simulink model "fas3dboc_2dexp_2019a"  (R2019a)
settings: Solver=ode4  StartTime=0.0  StopTime=20  FixedStep=0.1  RelTol=1e-3
libraries: sldrtlib x1
settings Model: Creator=star-laptop  LastModifiedBy=nochinese
settings DebuggingCC: UnconnectedInputMsg=none  UnconnectedOutputMsg=none  UnconnectedLineMsg=none

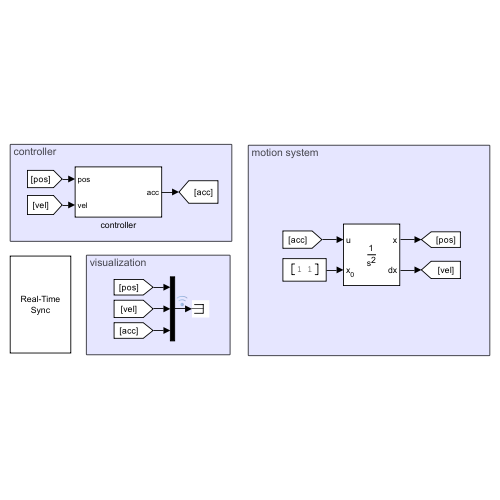
[thumbnail: Simulink's stored preview of the top-level diagram]
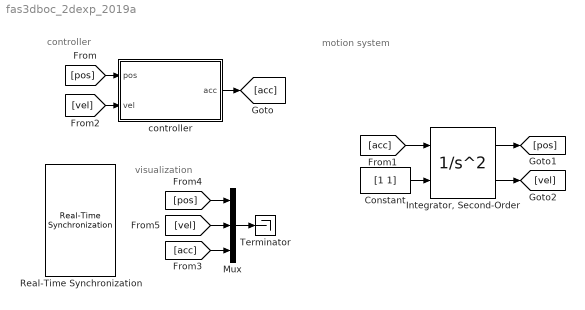
== system fas3dboc_2dexp_2019a ==
  note: motion system
  note: controller
  note: visualization
  Constant : Constant  Value=[1 1]
  "Integrator, Second-Order" : SecondOrderIntegrator  ICSourceX=external
  Mux : Mux  Inputs=3
  Real-Time Synchronization : sldrtlib/Real-Time Synchronization  SampleTime=0.1  MaxMissedTicks=10  ShowMissedTicks=off  YieldWhenWaiting=off
  Terminator : Terminator
  controller : Subsystem
  wires:
  controller/1(acc) -> [acc]
  [pos] -> controller/1(pos)
  "Integrator, Second-Order"/1 -> [pos]
  [acc] -> "Integrator, Second-Order"/1
  Constant/1 -> "Integrator, Second-Order"/2
  "Integrator, Second-Order"/2 -> [vel]
  [vel] -> controller/2(vel)
  Mux/1 -> Terminator/1
  [acc] -> Mux/3
  [pos] -> Mux/1
  [vel] -> Mux/2

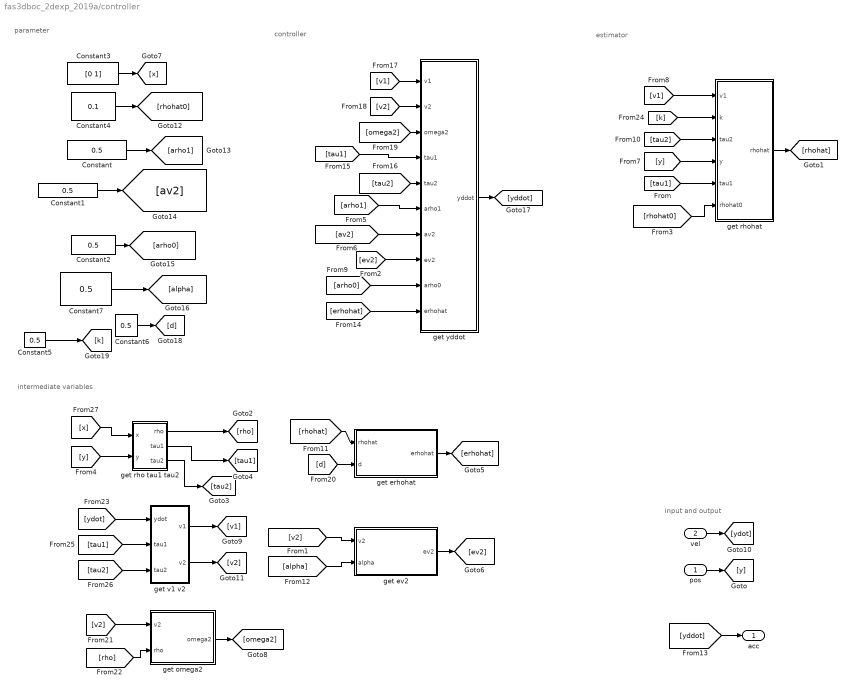
== system fas3dboc_2dexp_2019a/controller ==
  note: intermediate variables
  note: estimator
  note: controller
  note: parameter
  note: input and output
  pos : Inport
  vel : Inport  Port=2
  Constant{,1..2,5..7} (6 alike) : Constant  Value=0.5
  Constant3 : Constant  Value=[0 1]
  Constant4 : Constant  Value=0.1
  get erhohat : Subsystem
  get ev2 : Subsystem
  get omega2 : Subsystem
  get rho tau1 tau2 : Subsystem
  get rhohat : Subsystem
  get v1 v2 : Subsystem
  get yddot : Subsystem
  acc : Outport
  wires:
  pos/1 -> [y]
  [v1] -> get rhohat/1(v1)
  [tau2] -> get rhohat/3(tau2)
  [y] -> get rhohat/4(y)
  [tau1] -> get rhohat/5(tau1)
  get rhohat/1(rhohat) -> [rhohat]
  [rhohat] -> get erhohat/1(rhohat)
  get erhohat/1(erhohat) -> [erhohat]
  [v1] -> get yddot/1(v1)
  [v2] -> get yddot/2(v2)
  [omega2] -> get yddot/3(omega2)
  [tau1] -> get yddot/4(tau1)
  [tau2] -> get yddot/5(tau2)
  [ev2] -> get yddot/8(ev2)
  [erhohat] -> get yddot/10(erhohat)
  [v2] -> get ev2/1(v2)
  get ev2/1(ev2) -> [ev2]
  Constant3/1 -> [x]
  [v2] -> get omega2/1(v2)
  [rho] -> get omega2/2(rho)
  get omega2/1(omega2) -> [omega2]
  [ydot] -> get v1 v2/1(ydot)
  [tau1] -> get v1 v2/2(tau1)
  [tau2] -> get v1 v2/3(tau2)
  get v1 v2/1(v1) -> [v1]
  get v1 v2/2(v2) -> [v2]
  vel/1 -> [ydot]
  [x] -> get rho tau1 tau2/1(x)
  [y] -> get rho tau1 tau2/2(y)
  get rho tau1 tau2/1(rho) -> [rho]
  get rho tau1 tau2/2(tau1) -> [tau1]
  get rho tau1 tau2/3(tau2) -> [tau2]
  Constant4/1 -> [rhohat0]
  [rhohat0] -> get rhohat/6(rhohat0)
  Constant/1 -> [arho1]
  [arho1] -> get yddot/6(arho1)
  Constant1/1 -> [av2]
  [arho0] -> get yddot/9(arho0)
  Constant2/1 -> [arho0]
  [av2] -> get yddot/7(av2)
  [d] -> get erhohat/2(d)
  Constant6/1 -> [d]
  Constant7/1 -> [alpha]
  [alpha] -> get ev2/2(alpha)
  [yddot] -> acc/1
  get yddot/1(yddot) -> [yddot]
  Constant5/1 -> [k]
  [k] -> get rhohat/2(k)

== system fas3dboc_2dexp_2019a/controller/get erhohat ==
  rhohat : Inport
  d : Inport  Port=2
  Subtract : Sum  Inputs=+-
  erhohat : Outport
  wires:
  rhohat/1 -> Subtract/1
  d/1 -> Subtract/2
  Subtract/1 -> erhohat/1

== system fas3dboc_2dexp_2019a/controller/get ev2 ==
  v2 : Inport
  alpha : Inport  Port=2
  Subtract : Sum  Inputs=+-
  ev2 : Outport
  wires:
  v2/1 -> Subtract/1
  alpha/1 -> Subtract/2
  Subtract/1 -> ev2/1

== system fas3dboc_2dexp_2019a/controller/get omega2 ==
  v2 : Inport
  rho : Inport  Port=2
  Divide : Product  Inputs=*/
  omega2 : Outport
  wires:
  v2/1 -> Divide/1
  rho/1 -> Divide/2
  Divide/1 -> omega2/1

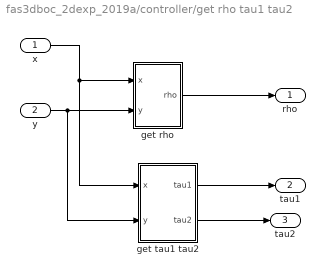
== system fas3dboc_2dexp_2019a/controller/get rho tau1 tau2 ==
  x : Inport
  y : Inport  Port=2
  get rho : Subsystem
  get tau1 tau2 : Subsystem
  rho : Outport
  tau1 : Outport  Port=2
  tau2 : Outport  Port=3
  wires:
  get tau1 tau2/2(tau2) -> tau2/1
  y/1 -> get tau1 tau2/2(y), get rho/2(y)
  get rho/1(rho) -> rho/1
  x/1 -> get tau1 tau2/1(x), get rho/1(x)
  get tau1 tau2/1(tau1) -> tau1/1

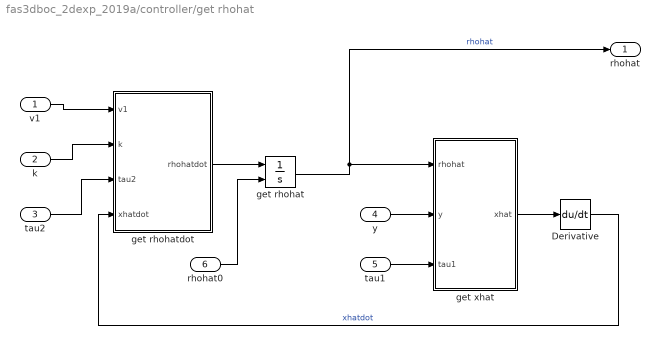
== system fas3dboc_2dexp_2019a/controller/get rhohat ==
  v1 : Inport
  k : Inport  Port=2
  tau2 : Inport  Port=3
  y : Inport  Port=4
  tau1 : Inport  Port=5
  rhohat0 : Inport  Port=6
  Derivative : Derivative
  get rhohat : Integrator  InitialConditionSource=external
  get rhohatdot : Subsystem
  get xhat : Subsystem
  rhohat : Outport
  wires:
  y/1 -> get xhat/2(y)
  get rhohat/1 -> rhohat/1, get xhat/1(rhohat)  "rhohat"
  get xhat/1(xhat) -> Derivative/1
  tau2/1 -> get rhohatdot/3(tau2)
  Derivative/1 -> get rhohatdot/4(xhatdot)  "xhatdot"
  get rhohatdot/1(rhohatdot) -> get rhohat/1
  v1/1 -> get rhohatdot/1(v1)
  tau1/1 -> get xhat/3(tau1)
  k/1 -> get rhohatdot/2(k)
  rhohat0/1 -> get rhohat/2

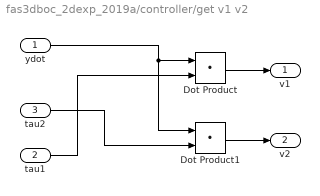
== system fas3dboc_2dexp_2019a/controller/get v1 v2 ==
  ydot : Inport
  tau1 : Inport  Port=2
  tau2 : Inport  Port=3
  Dot Product : DotProduct  InputSameDT=on  OutDataTypeStr=Inherit: Inherit via internal rule
  Dot Product1 : DotProduct  InputSameDT=on  OutDataTypeStr=Inherit: Inherit via internal rule
  v1 : Outport
  v2 : Outport  Port=2
  wires:
  ydot/1 -> Dot Product1/1, Dot Product/1
  Dot Product/1 -> v1/1
  Dot Product1/1 -> v2/1
  tau2/1 -> Dot Product1/2
  tau1/1 -> Dot Product/2

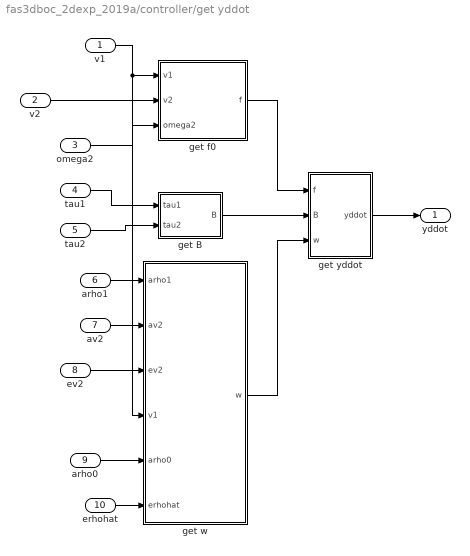
== system fas3dboc_2dexp_2019a/controller/get yddot ==
  v1 : Inport
  v2 : Inport  Port=2
  omega2 : Inport  Port=3
  tau1 : Inport  Port=4
  tau2 : Inport  Port=5
  arho1 : Inport  Port=6
  av2 : Inport  Port=7
  ev2 : Inport  Port=8
  arho0 : Inport  Port=9
  erhohat : Inport  Port=10
  get B : Subsystem
  get f0 : Subsystem
  get w : Subsystem
  get yddot : Subsystem
  yddot : Outport
  wires:
  tau1/1 -> get B/1(tau1)
  get B/1(B) -> get yddot/2(B)
  av2/1 -> get w/2(av2)
  ev2/1 -> get w/3(ev2)
  get yddot/1(yddot) -> yddot/1
  v1/1 -> get w/4(v1), get f0/1(v1)
  get w/1(w) -> get yddot/3(w)
  get f0/1(f) -> get yddot/1(f)
  v2/1 -> get f0/2(v2)
  omega2/1 -> get f0/3(omega2)
  tau2/1 -> get B/2(tau2)
  arho1/1 -> get w/1(arho1)
  erhohat/1 -> get w/6(erhohat)
  arho0/1 -> get w/5(arho0)

== system fas3dboc_2dexp_2019a/controller/get rho tau1 tau2/get rho ==
  note: $\rho=\|{\bf\it x}-{\bf\it y}\|$
  x : Inport
  y : Inport  Port=2
  Add : Sum  Inputs=+-
  Dot Product : DotProduct  InputSameDT=on  OutDataTypeStr=Inherit: Inherit via internal rule
  Sqrt : Sqrt  SaturateOnIntegerOverflow=on
  rho : Outport
  wires:
  Dot Product/1 -> Sqrt/1
  Add/1 -> Dot Product/2, Dot Product/1
  y/1 -> Add/2
  x/1 -> Add/1
  Sqrt/1 -> rho/1

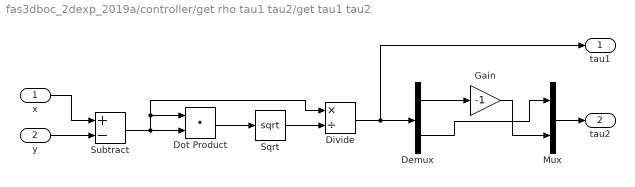
== system fas3dboc_2dexp_2019a/controller/get rho tau1 tau2/get tau1 tau2 ==
  x : Inport
  y : Inport  Port=2
  Demux : Demux  Outputs=2
  Divide : Product  Inputs=*/
  Dot Product : DotProduct  InputSameDT=on  OutDataTypeStr=Inherit: Inherit via internal rule
  Gain : Gain  Gain=-1
  Mux : Mux  Inputs=2
  Sqrt : Sqrt  SaturateOnIntegerOverflow=on
  Subtract : Sum  Inputs=+-
  tau1 : Outport
  tau2 : Outport  Port=2
  wires:
  Divide/1 -> tau1/1, Demux/1
  y/1 -> Subtract/2
  Sqrt/1 -> Divide/2
  Dot Product/1 -> Sqrt/1
  Gain/1 -> Mux/2
  Demux/2 -> Mux/1
  Subtract/1 -> Divide/1, Dot Product/1, Dot Product/2
  Demux/1 -> Gain/1
  Mux/1 -> tau2/1
  x/1 -> Subtract/1

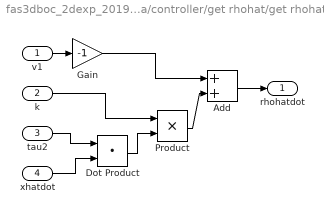
== system fas3dboc_2dexp_2019a/controller/get rhohat/get rhohatdot ==
  v1 : Inport
  k : Inport  Port=2
  tau2 : Inport  Port=3
  xhatdot : Inport  Port=4
  Add : Sum
  Dot Product : DotProduct  InputSameDT=on  OutDataTypeStr=Inherit: Inherit via internal rule
  Gain : Gain  Gain=-1
  Product : Product
  rhohatdot : Outport
  wires:
  tau2/1 -> Dot Product/1
  xhatdot/1 -> Dot Product/2
  Dot Product/1 -> Product/2
  k/1 -> Product/1
  v1/1 -> Gain/1
  Product/1 -> Add/2
  Gain/1 -> Add/1
  Add/1 -> rhohatdot/1

== system fas3dboc_2dexp_2019a/controller/get rhohat/get xhat ==
  rhohat : Inport
  y : Inport  Port=2
  tau1 : Inport  Port=3
  Add : Sum
  Product : Product
  xhat : Outport
  wires:
  rhohat/1 -> Product/1
  tau1/1 -> Product/2
  y/1 -> Add/1
  Product/1 -> Add/2
  Add/1 -> xhat/1

== system fas3dboc_2dexp_2019a/controller/get yddot/get B ==
  tau1 : Inport
  tau2 : Inport  Port=2
  Gain : Gain  Gain=-1
  Matrix Concatenate : Concatenate  Mode=Multidimensional array  ConcatenateDimension=2
  Transpose : Math  Operator=transpose  SaturateOnIntegerOverflow=on
  B : Outport
  wires:
  tau1/1 -> Gain/1
  Gain/1 -> Matrix Concatenate/1
  tau2/1 -> Matrix Concatenate/2
  Matrix Concatenate/1 -> Transpose/1
  Transpose/1 -> B/1

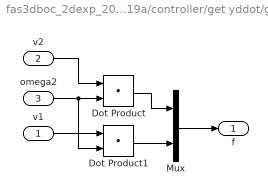
== system fas3dboc_2dexp_2019a/controller/get yddot/get f0 ==
  v1 : Inport
  v2 : Inport  Port=2
  omega2 : Inport  Port=3
  Dot Product : DotProduct  InputSameDT=on  OutDataTypeStr=Inherit: Inherit via internal rule
  Dot Product1 : DotProduct  InputSameDT=on  OutDataTypeStr=Inherit: Inherit via internal rule
  Mux : Mux  Inputs=2
  f : Outport
  wires:
  Dot Product1/1 -> Mux/2
  v2/1 -> Dot Product/1
  Mux/1 -> f/1
  omega2/1 -> Dot Product1/2, Dot Product/2
  v1/1 -> Dot Product1/1
  Dot Product/1 -> Mux/1

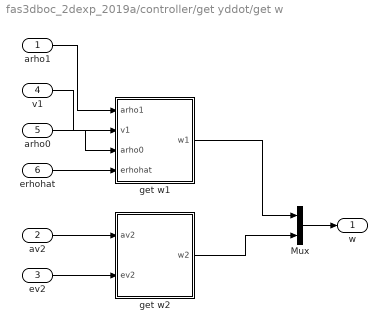
== system fas3dboc_2dexp_2019a/controller/get yddot/get w ==
  arho1 : Inport
  av2 : Inport  Port=2
  ev2 : Inport  Port=3
  v1 : Inport  Port=4
  arho0 : Inport  Port=5
  erhohat : Inport  Port=6
  Mux : Mux  Inputs=2
  get w1 : Subsystem
  get w2 : Subsystem
  w : Outport
  wires:
  get w1/1(w1) -> Mux/1
  Mux/1 -> w/1
  av2/1 -> get w2/1(av2)
  ev2/1 -> get w2/2(ev2)
  erhohat/1 -> get w1/4(erhohat)
  arho0/1 -> get w1/3(arho0)
  v1/1 -> get w1/2(v1)
  arho1/1 -> get w1/1(arho1)
  get w2/1(w2) -> Mux/2

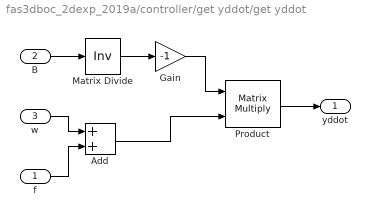
== system fas3dboc_2dexp_2019a/controller/get yddot/get yddot ==
  f : Inport
  B : Inport  Port=2
  w : Inport  Port=3
  Add : Sum
  Gain : Gain  Gain=-1
  Matrix Divide : Product  Inputs=/  Multiplication=Matrix(*)
  Product : Product  Multiplication=Matrix(*)
  yddot : Outport
  wires:
  B/1 -> Matrix Divide/1
  Matrix Divide/1 -> Gain/1
  w/1 -> Add/1
  f/1 -> Add/2
  Gain/1 -> Product/1
  Add/1 -> Product/2
  Product/1 -> yddot/1

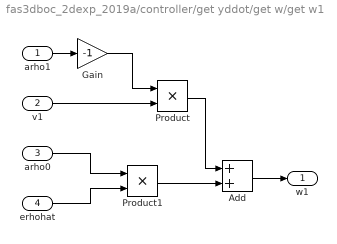
== system fas3dboc_2dexp_2019a/controller/get yddot/get w/get w1 ==
  arho1 : Inport
  v1 : Inport  Port=2
  arho0 : Inport  Port=3
  erhohat : Inport  Port=4
  Add : Sum
  Gain : Gain  Gain=-1
  Product : Product
  Product1 : Product
  w1 : Outport
  wires:
  arho1/1 -> Gain/1
  Gain/1 -> Product/1
  v1/1 -> Product/2
  arho0/1 -> Product1/1
  erhohat/1 -> Product1/2
  Product1/1 -> Add/2
  Product/1 -> Add/1
  Add/1 -> w1/1

== system fas3dboc_2dexp_2019a/controller/get yddot/get w/get w2 ==
  av2 : Inport
  ev2 : Inport  Port=2
  Product1 : Product
  w2 : Outport
  wires:
  Product1/1 -> w2/1
  ev2/1 -> Product1/2
  av2/1 -> Product1/1
